simulink model "RLModel"  (R2024b)
settings: Solver=VariableStepAuto  StartTime=0.0  StopTime=Tf  RelTol=1e-3  AbsTol=1e-3  EnableMultiTasking=on
InitFcn:
  | ModelParameters;
values from neighbouring files (symbols this model uses):
  foot_height = 0.05    [ModelParameters.m]
  foot_length = 0.3    [ModelParameters.m]
  foot_width = 0.2    [ModelParameters.m]
  init_height = plane_height/2 + foot_height + shank_height + thigh_height + 0.5*torso_height    (= 1.65)    [ModelParameters.m]
  left = [0,          0,          0]    [ModelParameters.m]
  max_torque = 1000    [ModelParameters.m]
  plane_height = 0.2    [ModelParameters.m]
  right = [0,          0,          0]    [ModelParameters.m]
  shank_height = 0.5    [ModelParameters.m]
  shank_length = 0.2    [ModelParameters.m]
  shank_width = 0.2    [ModelParameters.m]
  Tf = 10.0    (= 10)    [ModelParameters.m]
  thigh_height = 0.5    [ModelParameters.m]
  thigh_length = 0.2    [ModelParameters.m]
  thigh_width = 0.2    [ModelParameters.m]
  torso_height = 1.0    (= 1)    [ModelParameters.m]
  torso_length = 0.2    [ModelParameters.m]
  torso_width = 0.5    [ModelParameters.m]
  Ts = 0.025    [ModelParameters.m]
undefined symbols (not defined in the file or in its folder): X, Y, Z
libraries: sm_lib x62, nesl_utility x25, rllib x1, simulink x1
(part 1 of 3)
settings Model: Creator=anbes  LastModifiedBy=anbes
settings SolverCC: AutoScaleAbsTol=off  AlgebraicLoopSolver=TrustRegion  MaxZcPerStep=1
settings DataIOCC: LimitDataPoints=on  MaxDataPoints=10000
settings OptimizationCC: ReuseModelBlockBuffer=off  LifeSpan=inf
settings DebuggingCC: UnconnectedInputMsg=warning  UnconnectedOutputMsg=warning  UnconnectedLineMsg=warning  AllowSymbolicDim=off  SubsystemReferenceDiagnosticForUnitTest=warning  SFUnexpectedBacktrackingDiag=warning  SFNoUnconditionalDefaultTransitionDiag=warning  SFExecutionAtInitializationDiag=none  ArithmeticOperatorsInVariantConditions=warning
settings ModelReferenceCC: EnableRefExpFcnMdlSchedulingChecks=on
settings SFSimCC: SimUseLocalCustomCode=off  CustomCodeUndefinedFunction=UseInterfaceOnly
settings RTWCC: RTWUseLocalCustomCode=off  GPUComputeCapability=3.5  DLArmComputeVersion=19.05
settings CodeAppCC: StateflowObjectComments=on
settings GRTTargetCC: TargetLangStandard=C89/C90 (ANSI)
settings ConfigComp: CovMetricSettings=dw  CovSaveCumulativeToWorkspaceVar=on  CovSaveSingleToWorkspaceVar=on  CovExternalEMLEnable=off  CovSFcnEnable=off
settings SimscapeCC: SimscapeLogType=all  SimscapeLogSimulationStatistics=on  SimscapeLogDataHistory=10000

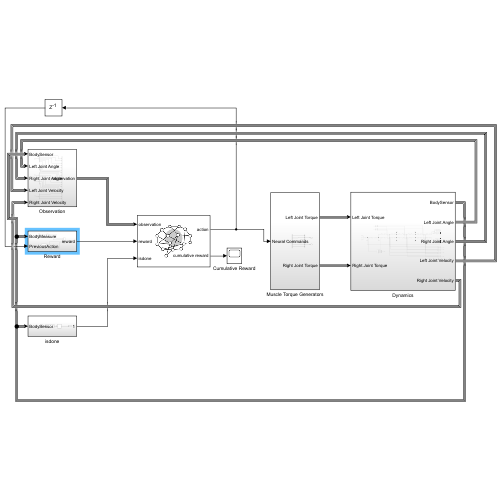
[thumbnail: Simulink's stored preview of the top-level diagram]
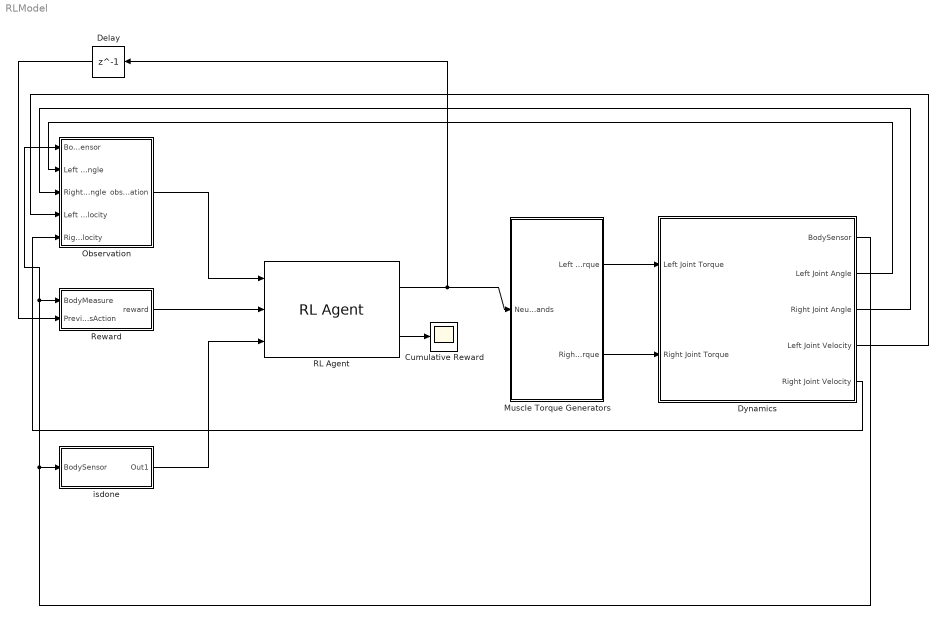
== system RLModel ==
  Cumulative Reward : Scope
  Delay : Delay  DelayLength=1  InitialCondition=0
  Dynamics : Subsystem
  Muscle Torque Generators : Subsystem
  Observation : Subsystem
  RL Agent : rllib/RL Agent  Agent=agent  ExternalActionAsInput=off  ProvideLastAction=off  ProvideCumRwd=on  TreatAsDirectFeedthrough=on  UseStrictObservationDataTypes=off
  Reward : Subsystem
  isdone : Subsystem
  wires:
  Muscle Torque Generators/1(Left Joint Torque) -> Dynamics/1(Left Joint Torque)
  Muscle Torque Generators/2(Right Joint Torque) -> Dynamics/2(Right Joint Torque)
  RL Agent/1 -> Delay/1, Muscle Torque Generators/1(Neural Commands)
  Dynamics/1(BodySensor) -> Observation/1(BodySensor), Reward/1(BodyMeasure), isdone/1(BodySensor)
  isdone/1(Out1) -> RL Agent/3
  Delay/1 -> Reward/2(PreviousAction)
  Reward/1(reward) -> RL Agent/2
  Dynamics/2(Left Joint Angle) -> Observation/2(Left Joint Angle)
  Dynamics/3(Right Joint Angle) -> Observation/3(Right Joint Angle)
  Dynamics/4(Left Joint Velocity) -> Observation/4(Left Joint Velocity)
  Observation/1(observation) -> RL Agent/1
  RL Agent/2 -> Cumulative Reward/1
  Dynamics/5(Right Joint Velocity) -> Observation/5(Right Joint Velocity)
